simulink model "sim_SS"  (R2021a)
settings: Solver=VariableStepAuto  StartTime=0.0  StopTime=50  MaxStep=0.02  RelTol=1e-3  AbsTol=1e-3
values from neighbouring files (symbols this model uses):
  A = [0    1     0    0 ... (first row only)    [state_space_matrices.m]
  b = 0.5    [system_params.m]
  B = [0 0;1/m1 0;0 0;0 1/m2]    [state_space_matrices.m]
  C_1 = eye(4)    [state_space_matrices.m]
  C_2 = [1 0 0 0]    [state_space_matrices.m]
  C_3 = [0 0 1 0]    [state_space_matrices.m]
  Kf_1 = lqr(A',C_1',Q,R)'    [state_space_matrices.m]
  Kf_2 = lqr(A',C_2',Q,R)'    [state_space_matrices.m]
  Kf_3 = lqr(A',C_3',Q,R)'    [state_space_matrices.m]
  Ts = 0.01    [system_params.m]
libraries: fl_lib x13, nesl_utility x7, simulink x6
settings Model: Creator=husse  LastModifiedBy=husse
settings SolverCC: AutoScaleAbsTol=off  AlgebraicLoopSolver=TrustRegion
settings DebuggingCC: SymbolicDimsDataTypeCodeGenerationDiagnostic=none  SFMachineParentedDataDiag=warning
settings SFSimCC: CustomCodeUndefinedFunction=UseInterfaceOnly
settings SimscapeCC: SimscapeLogType=all  SimscapeLogSimulationStatistics=on  SimscapeLogDataHistory=10000

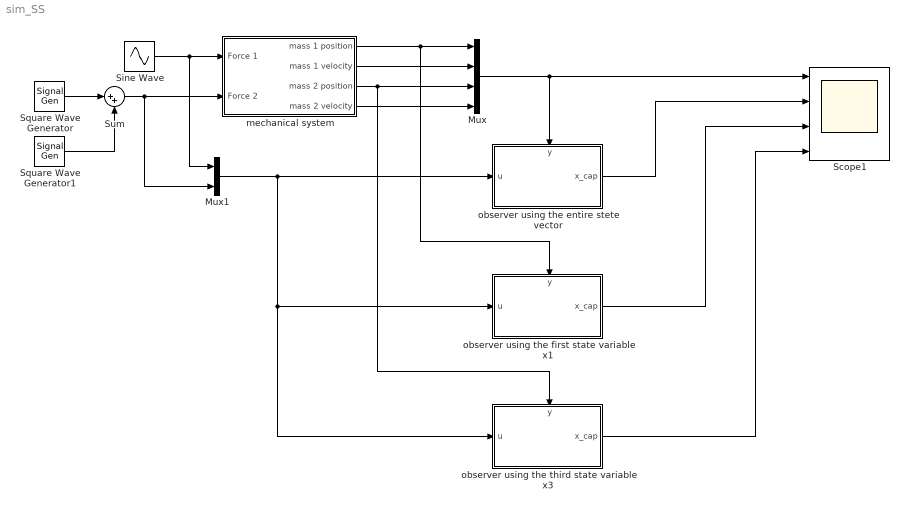
== system sim_SS ==
  Mux : Mux
  Mux1 : Mux  Inputs=2
  Scope1 : Scope  NumInputPorts=4
  Sine Wave : Sin  SampleTime=0
  Square Wave Generator : SignalGenerator  WaveForm=square  Units=rad/sec
  Square Wave Generator1 : SignalGenerator  WaveForm=sawtooth  Units=rad/sec
  Sum : Sum  Inputs=|++
  mechanical system : Subsystem
  observer using the entire stete vector : Subsystem
      settings: PortSchema="{\"entries\":[{\"content\":{\"sides\":[{\"content\":{\"connectorIds\":[\"In1\"]},\"type\":\"ConnectorPlacement.EquallySpacedRectSide\",\"uuid\":\"986d422d-b8ff-4d9a-baf2-00a8ac9f9019\"},{\"content\":{\"connectorIds\":[\"Out1\"],\"side\":\"RIGHT\"},\"type\":\"ConnectorPlacement.EquallySpacedRectSide\",\"uuid\":\"59e96993-3a48-4151-9be3-a9dc09e1e33d\"},{\"content\":{\"connectorIds\":[\"In2\"],\"side\":\"TOP\"},\"type\":\"ConnectorPlacement.EquallySpacedRectSide\",\"uuid\":\"13ba996f-1b17-4586-8eaf-63e69bc07399\"}]},\"type\":\"ConnectorPlacement.EquallySpacedConnector\",\"uuid\":\"b109a439-7035-48cd-b1f6-10e4a3832946\"}],\"packageUris\":[\"http://schema.mathworks.com/mf0/Connector/R2020b\"],\"version\":\"1.0\"}"
  observer using the first state variable x1 : Subsystem
      settings: PortSchema="{\"entries\":[{\"content\":{\"sides\":[{\"content\":{\"connectorIds\":[\"In1\"]},\"type\":\"ConnectorPlacement.EquallySpacedRectSide\",\"uuid\":\"986d422d-b8ff-4d9a-baf2-00a8ac9f9019\"},{\"content\":{\"connectorIds\":[\"Out1\"],\"side\":\"RIGHT\"},\"type\":\"ConnectorPlacement.EquallySpacedRectSide\",\"uuid\":\"59e96993-3a48-4151-9be3-a9dc09e1e33d\"},{\"content\":{\"connectorIds\":[\"In2\"],\"side\":\"TOP\"},\"type\":\"ConnectorPlacement.EquallySpacedRectSide\",\"uuid\":\"13ba996f-1b17-4586-8eaf-63e69bc07399\"}]},\"type\":\"ConnectorPlacement.EquallySpacedConnector\",\"uuid\":\"b109a439-7035-48cd-b1f6-10e4a3832946\"}],\"packageUris\":[\"http://schema.mathworks.com/mf0/Connector/R2020b\"],\"version\":\"1.0\"}"
  observer using the third state variable x3 : Subsystem
      settings: PortSchema="{\"entries\":[{\"content\":{\"sides\":[{\"content\":{\"connectorIds\":[\"In1\"]},\"type\":\"ConnectorPlacement.EquallySpacedRectSide\",\"uuid\":\"986d422d-b8ff-4d9a-baf2-00a8ac9f9019\"},{\"content\":{\"connectorIds\":[\"Out1\"],\"side\":\"RIGHT\"},\"type\":\"ConnectorPlacement.EquallySpacedRectSide\",\"uuid\":\"59e96993-3a48-4151-9be3-a9dc09e1e33d\"},{\"content\":{\"connectorIds\":[\"In2\"],\"side\":\"TOP\"},\"type\":\"ConnectorPlacement.EquallySpacedRectSide\",\"uuid\":\"13ba996f-1b17-4586-8eaf-63e69bc07399\"}]},\"type\":\"ConnectorPlacement.EquallySpacedConnector\",\"uuid\":\"b109a439-7035-48cd-b1f6-10e4a3832946\"}],\"packageUris\":[\"http://schema.mathworks.com/mf0/Connector/R2020b\"],\"version\":\"1.0\"}"
  wires:
  Sine Wave/1 -> Mux1/1, mechanical system/1(Force 1)
  mechanical system/1(mass 1 position) -> observer using the first state variable x1/2(y), Mux/1
  mechanical system/2(mass 1 velocity) -> Mux/2
  mechanical system/3(mass 2 position) -> Mux/3, observer using the third state variable x3/2(y)
  mechanical system/4(mass 2 velocity) -> Mux/4
  Mux/1 -> observer using the entire stete vector/2(y), Scope1/1
  Mux1/1 -> observer using the third state variable x3/1(u), observer using the first state variable x1/1(u), observer using the entire stete vector/1(u)
  observer using the entire stete vector/1(x_cap) -> Scope1/2
  observer using the first state variable x1/1(x_cap) -> Scope1/3
  observer using the third state variable x3/1(x_cap) -> Scope1/4
  Square Wave Generator/1 -> Sum/1
  Sum/1 -> Mux1/2, mechanical system/2(Force 2)
  Square Wave Generator1/1 -> Sum/2

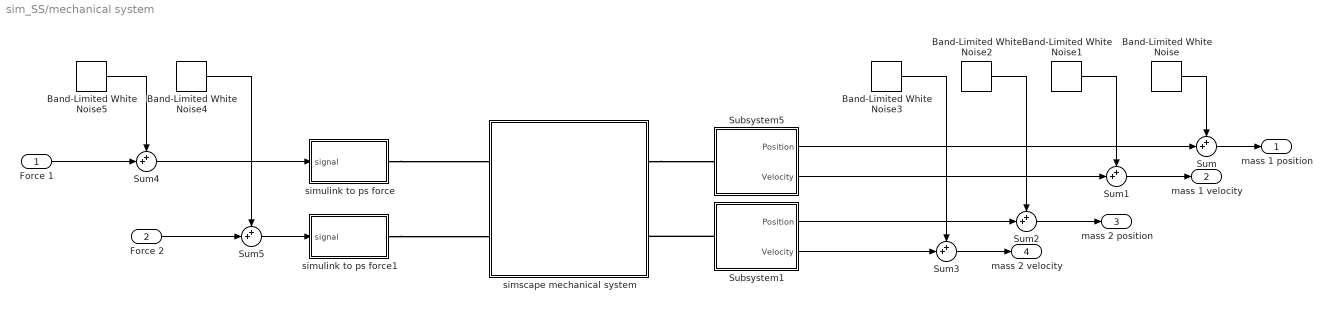
== system sim_SS/mechanical system ==
  Force 1 : Inport
  Force 2 : Inport  Port=2
  Band-Limited White Noise : simulink/Sources/Band-Limited White Noise  Cov=n  Ts=Ts  seed=[23341]
  Band-Limited White Noise1 : simulink/Sources/Band-Limited White Noise  Cov=n  Ts=Ts  seed=[23345]
  Band-Limited White Noise2 : simulink/Sources/Band-Limited White Noise  Cov=n  Ts=Ts  seed=[28341]
  Band-Limited White Noise3 : simulink/Sources/Band-Limited White Noise  Cov=n  Ts=Ts  seed=[23391]
  Band-Limited White Noise4 : simulink/Sources/Band-Limited White Noise  Cov=n  Ts=Ts  seed=[23391]
  Band-Limited White Noise5 : simulink/Sources/Band-Limited White Noise  Cov=n  Ts=Ts  seed=[23391]
  Subsystem1 : Subsystem
  Subsystem5 : Subsystem
  Sum{,1..5} (6 alike) : Sum  Inputs=++|
  simscape mechanical system : Subsystem
  simulink to ps force : Subsystem
  simulink to ps force1 : Subsystem
  mass 1 position : Outport
  mass 1 velocity : Outport  Port=2
  mass 2 position : Outport  Port=3
  mass 2 velocity : Outport  Port=4
  wires:
  Subsystem5/1(Position) -> Sum/2
  Sum/1 -> mass 1 position/1
  Subsystem5/2(Velocity) -> Sum1/2
  Sum1/1 -> mass 1 velocity/1
  Sum2/1 -> mass 2 position/1
  Subsystem1/1(Position) -> Sum2/2
  Sum3/1 -> mass 2 velocity/1
  Subsystem1/2(Velocity) -> Sum3/2
  Band-Limited White Noise/1 -> Sum/1
  Band-Limited White Noise1/1 -> Sum1/1
  Band-Limited White Noise2/1 -> Sum2/1
  Band-Limited White Noise3/1 -> Sum3/1
  Force 1/1 -> Sum4/2
  Sum4/1 -> simulink to ps force/1(signal)
  Sum5/1 -> simulink to ps force1/1(signal)
  Force 2/1 -> Sum5/2
  Band-Limited White Noise5/1 -> Sum4/1
  Band-Limited White Noise4/1 -> Sum5/1
  connections:
  simulink to ps force1/RConn1 -- simscape mechanical system/LConn2
  Subsystem1/LConn1 -- simscape mechanical system/RConn2
  simscape mechanical system/RConn1 -- Subsystem5/LConn1
  simulink to ps force/RConn1 -- simscape mechanical system/LConn1

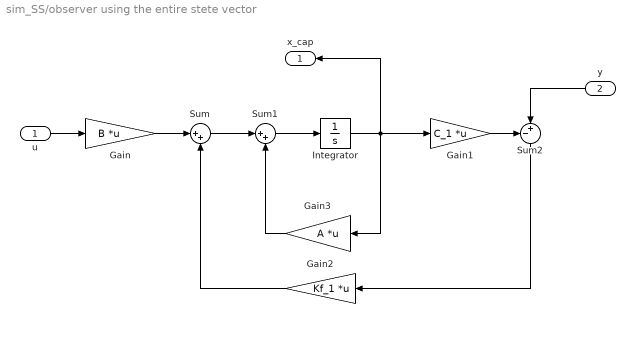
== system sim_SS/observer using the entire stete vector ==
  u : Inport
  y : Inport  Port=2
  Gain : Gain  Gain=B  Multiplication=Matrix(K*u)
  Gain1 : Gain  Gain=C_1  Multiplication=Matrix(K*u)
  Gain2 : Gain  Gain=Kf_1  Multiplication=Matrix(K*u)
  Gain3 : Gain  Gain=A  Multiplication=Matrix(K*u)
  Integrator : Integrator  InitialCondition=[0 0 0 0]
  Sum : Sum  Inputs=|++
  Sum1 : Sum  Inputs=|++
  Sum2 : Sum  Inputs=-+|
  x_cap : Outport
  wires:
  Gain2/1 -> Sum/2
  Sum2/1 -> Gain2/1
  Gain1/1 -> Sum2/1
  Integrator/1 -> x_cap/1, Gain3/1, Gain1/1
  Sum/1 -> Sum1/1
  Sum1/1 -> Integrator/1
  Gain3/1 -> Sum1/2
  Gain/1 -> Sum/1
  y/1 -> Sum2/2
  u/1 -> Gain/1

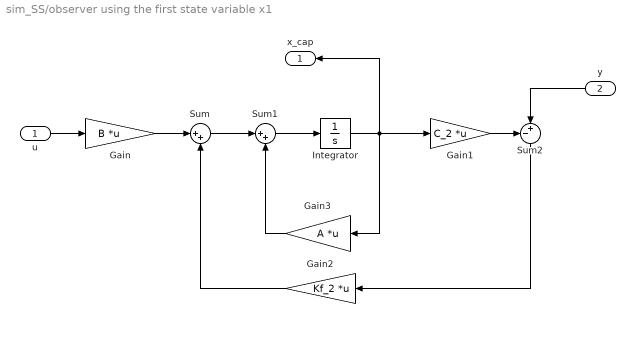
== system sim_SS/observer using the first state variable x1 ==
  u : Inport
  y : Inport  Port=2
  Gain : Gain  Gain=B  Multiplication=Matrix(K*u)
  Gain1 : Gain  Gain=C_2  Multiplication=Matrix(K*u)
  Gain2 : Gain  Gain=Kf_2  Multiplication=Matrix(K*u)
  Gain3 : Gain  Gain=A  Multiplication=Matrix(K*u)
  Integrator : Integrator
  Sum : Sum  Inputs=|++
  Sum1 : Sum  Inputs=|++
  Sum2 : Sum  Inputs=-+|
  x_cap : Outport
  wires:
  u/1 -> Gain/1
  y/1 -> Sum2/2
  Gain/1 -> Sum/1
  Gain3/1 -> Sum1/2
  Sum1/1 -> Integrator/1
  Sum/1 -> Sum1/1
  Integrator/1 -> Gain1/1, Gain3/1, x_cap/1
  Gain1/1 -> Sum2/1
  Sum2/1 -> Gain2/1
  Gain2/1 -> Sum/2

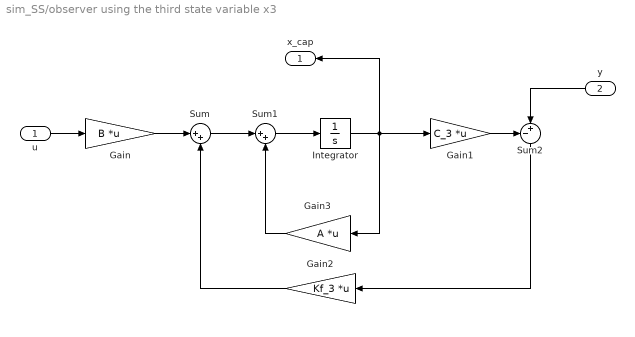
== system sim_SS/observer using the third state variable x3 ==
  u : Inport
  y : Inport  Port=2
  Gain : Gain  Gain=B  Multiplication=Matrix(K*u)
  Gain1 : Gain  Gain=C_3  Multiplication=Matrix(K*u)
  Gain2 : Gain  Gain=Kf_3  Multiplication=Matrix(K*u)
  Gain3 : Gain  Gain=A  Multiplication=Matrix(K*u)
  Integrator : Integrator
  Sum : Sum  Inputs=|++
  Sum1 : Sum  Inputs=|++
  Sum2 : Sum  Inputs=-+|
  x_cap : Outport
  wires:
  Gain2/1 -> Sum/2
  Sum2/1 -> Gain2/1
  Gain1/1 -> Sum2/1
  Integrator/1 -> x_cap/1, Gain3/1, Gain1/1
  Sum/1 -> Sum1/1
  Sum1/1 -> Integrator/1
  Gain3/1 -> Sum1/2
  Gain/1 -> Sum/1
  y/1 -> Sum2/2
  u/1 -> Gain/1

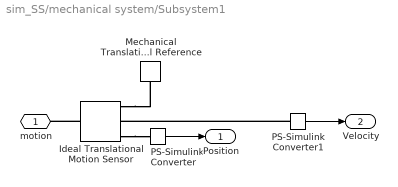
== system sim_SS/mechanical system/Subsystem1 ==
  Ideal Translational Motion Sensor : fl_lib/Mechanical/Mechanical Sensors/Ideal Translational Motion Sensor  offset=0 m
  Mechanical Translational Reference : fl_lib/Mechanical/Translational Elements/Mechanical Translational Reference
  PS-Simulink Converter : nesl_utility/PS-Simulink Converter  PhysicalDomain=network_engine_domain  SubClassName=ps_output  LeftPortType=input  RightPortType=output  PseudoPeriodic=off  Frequencies=[]  Unit=inherit  AffineConversion=off
      settings: SourceProductBaseCode=PW,SS
  PS-Simulink Converter1 : nesl_utility/PS-Simulink Converter  PhysicalDomain=network_engine_domain  SubClassName=ps_output  LeftPortType=input  RightPortType=output  PseudoPeriodic=off  Frequencies=[]  Unit=inherit  AffineConversion=off
      settings: SourceProductBaseCode=PW,SS
  motion : PMIOPort  Side=Left
  Position : Outport
  Velocity : Outport  Port=2
  wires:
  PS-Simulink Converter1/1 -> Velocity/1
  PS-Simulink Converter/1 -> Position/1
  connections:
  Ideal Translational Motion Sensor/LConn1 -- motion/RConn1
  Ideal Translational Motion Sensor/RConn3 -- PS-Simulink Converter/LConn1
  PS-Simulink Converter1/LConn1 -- Ideal Translational Motion Sensor/RConn2
  Ideal Translational Motion Sensor/RConn1 -- Mechanical Translational Reference/LConn1

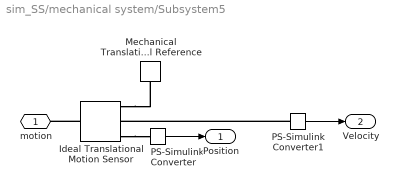
== system sim_SS/mechanical system/Subsystem5 ==
  Ideal Translational Motion Sensor : fl_lib/Mechanical/Mechanical Sensors/Ideal Translational Motion Sensor  offset=0 m
  Mechanical Translational Reference : fl_lib/Mechanical/Translational Elements/Mechanical Translational Reference
  PS-Simulink Converter : nesl_utility/PS-Simulink Converter  PhysicalDomain=network_engine_domain  SubClassName=ps_output  LeftPortType=input  RightPortType=output  PseudoPeriodic=off  Frequencies=[]  Unit=inherit  AffineConversion=off
      settings: SourceProductBaseCode=PW,SS
  PS-Simulink Converter1 : nesl_utility/PS-Simulink Converter  PhysicalDomain=network_engine_domain  SubClassName=ps_output  LeftPortType=input  RightPortType=output  PseudoPeriodic=off  Frequencies=[]  Unit=inherit  AffineConversion=off
      settings: SourceProductBaseCode=PW,SS
  motion : PMIOPort  Side=Left
  Position : Outport
  Velocity : Outport  Port=2
  wires:
  PS-Simulink Converter/1 -> Position/1
  PS-Simulink Converter1/1 -> Velocity/1
  connections:
  Ideal Translational Motion Sensor/RConn1 -- Mechanical Translational Reference/LConn1
  PS-Simulink Converter1/LConn1 -- Ideal Translational Motion Sensor/RConn2
  Ideal Translational Motion Sensor/RConn3 -- PS-Simulink Converter/LConn1
  Ideal Translational Motion Sensor/LConn1 -- motion/RConn1

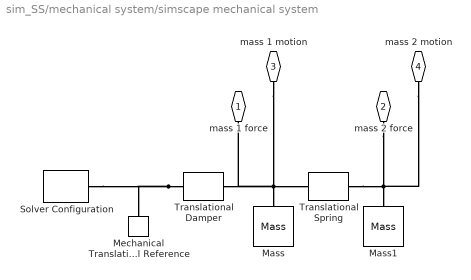
== system sim_SS/mechanical system/simscape mechanical system ==
  Mass : fl_lib/Mechanical/Translational Elements/Mass  mass=m1 kg  num_ports=foundation.enum.numPorts2.one  v_specify=off  v_priority=High  v=0 m/s  v_nominal_specify=off  v_nominal_unit=m/s  v_nominal_value=1  f_specify=off  f_priority=None  f=0 N  f_nominal_specify=off  f_nominal_unit=N  f_nominal_value=1
  Mass1 : fl_lib/Mechanical/Translational Elements/Mass  mass=m2 kg  num_ports=foundation.enum.numPorts2.one  v_specify=off  v_priority=High  v=0 m/s  v_nominal_specify=off  v_nominal_unit=m/s  v_nominal_value=1  f_specify=off  f_priority=None  f=0 N  f_nominal_specify=off  f_nominal_unit=N  f_nominal_value=1
  Mechanical Translational Reference : fl_lib/Mechanical/Translational Elements/Mechanical Translational Reference
  Solver Configuration : nesl_utility/Solver Configuration  PhysicalDomain=network_engine_domain  SubClassName=solver  LeftPortType=input  RightPortType=generic  Tones=[]  Harmonics=[]  SimulateNoise=off  Profile=off  UseLocalSampling=off  EnableSwitchedLinearOptims=on  FrequencyDomain=off  UseCCode=off  RelTol=0.001  AbsTol=1e-06  MinStep=1e-09  ToWorkspace=off  RevertToSquareIcSolve=off  NumHomotopyIterations=100  PhasorMode=off  PhasorModeNumHarmonics=1  DoDC=off  ResidualTolerance=1e-09  UseLocalSolver=off  LocalSolverChoice=NE_BACKWARD_EULER_ADVANCER  LocalSolverSampleTime=0.001  DoFixedCost=off  MaxNonlinIter=3  MaxModeIter=2  ComputeImpulses=off  ImpulseIterations=2  LinearAlgebra=auto  EquationFormulation=NE_TIME_EF  DelaysMemoryBudget=1024  AutomaticFiltering=on  FilteringTimeConstant=0.001  PartitionStorageMethod=AS_NEEDED  PartitionMemoryBudget=1024  PartitionMethod=ROBUST
      settings: SourceProductBaseCode=PW,SS
  Translational Damper : fl_lib/Mechanical/Translational Elements/Translational Damper  D=b N/(m/s)  v_specify=off  v_priority=None  v=0 m/s  v_nominal_specify=off  v_nominal_unit=m/s  v_nominal_value=1  f_specify=off  f_priority=None  f=0 N  f_nominal_specify=off  f_nominal_unit=N  f_nominal_value=1
  Translational Spring : fl_lib/Mechanical/Translational Elements/Translational Spring  spr_rate=k N/m  v_specify=off  v_priority=None  v=0 m/s  v_nominal_specify=off  v_nominal_unit=m/s  v_nominal_value=1  f_specify=off  f_priority=None  f=0 N  f_nominal_specify=off  f_nominal_unit=N  f_nominal_value=1  x_specify=off  x_priority=High  x=0 m  x_nominal_specify=off  x_nominal_unit=m  x_nominal_value=1
  mass 1 force : PMIOPort  Side=Left
  mass 2 force : PMIOPort  Port=2  Side=Left
  mass 1 motion : PMIOPort  Port=3  Side=Right
  mass 2 motion : PMIOPort  Port=4  Side=Right
  connections:
  Translational Damper/LConn1 -- Mechanical Translational Reference/LConn1 -- Solver Configuration/RConn1
  mass 2 motion/RConn1 -- Translational Spring/RConn1 -- Mass1/LConn1 -- mass 2 force/RConn1
  mass 1 motion/RConn1 -- Mass/LConn1 -- Translational Spring/LConn1 -- mass 1 force/RConn1 -- Translational Damper/RConn1

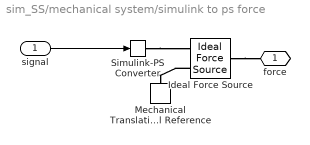
== system sim_SS/mechanical system/simulink to ps force ==
  signal : Inport
  Ideal Force Source : fl_lib/Mechanical/Mechanical Sources/Ideal Force Source
  Mechanical Translational Reference : fl_lib/Mechanical/Translational Elements/Mechanical Translational Reference
  Simulink-PS Converter : nesl_utility/Simulink-PS Converter  PhysicalDomain=network_engine_domain  SubClassName=ps_input  LeftPortType=input  RightPortType=output  PseudoPeriodic=off  Frequencies=[]  NoiseDistribution=none  NoiseParameters=[]  Unit=1  AffineConversion=off  FilteringAndDerivatives=provide  SimscapeFilterOrder=1  InputFilterTimeConstant=0.001  UdotUserProvided=0
      settings: SourceProductBaseCode=PW,SS
  force : PMIOPort  Side=Right
  wires:
  signal/1 -> Simulink-PS Converter/1
  connections:
  Ideal Force Source/LConn1 -- force/RConn1
  Simulink-PS Converter/RConn1 -- Ideal Force Source/RConn1
  Ideal Force Source/RConn2 -- Mechanical Translational Reference/LConn1

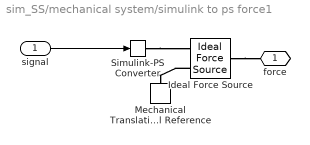
== system sim_SS/mechanical system/simulink to ps force1 ==
  signal : Inport
  Ideal Force Source : fl_lib/Mechanical/Mechanical Sources/Ideal Force Source
  Mechanical Translational Reference : fl_lib/Mechanical/Translational Elements/Mechanical Translational Reference
  Simulink-PS Converter : nesl_utility/Simulink-PS Converter  PhysicalDomain=network_engine_domain  SubClassName=ps_input  LeftPortType=input  RightPortType=output  PseudoPeriodic=off  Frequencies=[]  NoiseDistribution=none  NoiseParameters=[]  Unit=1  AffineConversion=off  FilteringAndDerivatives=provide  SimscapeFilterOrder=1  InputFilterTimeConstant=0.001  UdotUserProvided=0
      settings: SourceProductBaseCode=PW,SS
  force : PMIOPort  Side=Right
  wires:
  signal/1 -> Simulink-PS Converter/1
  connections:
  Ideal Force Source/RConn2 -- Mechanical Translational Reference/LConn1
  Simulink-PS Converter/RConn1 -- Ideal Force Source/RConn1
  Ideal Force Source/LConn1 -- force/RConn1
